simulink model "SM_FO_Simulink"  (R2025a)
settings: Solver=VariableStepAuto  StartTime=0.0  StopTime=10.0  RelTol=1e-3
settings Model: Creator=ryanjing  LastModifiedBy=ryanjing

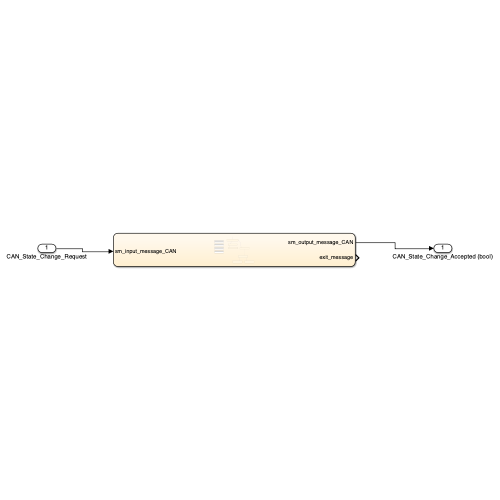
[thumbnail: Simulink's stored preview of the top-level diagram]
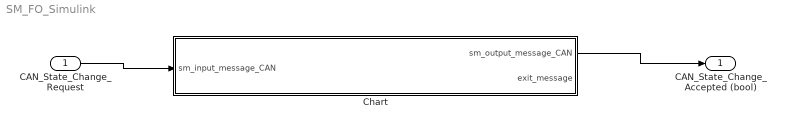
== system SM_FO_Simulink ==
  CAN_State_Change_Request : Inport
  Chart : Stateflow chart  TreatAsAtomicUnit=on
  CAN_State_Change_Accepted (bool) : Outport
  wires:
  CAN_State_Change_Request/1 -> Chart/1(sm_input_message_CAN)
  Chart/1(sm_output_message_CAN) -> CAN_State_Change_Accepted (bool)/1

== stateflow chart SM_FO_Simulink/Chart ==
  state Entry_State
    entry:
    parsed_message = parseCANMessage(sm_input_message_CAN);
  state Init_State
    entry:
    entry_status = SMFO_Init(sm_input_message_CAN);
  state Started_State
    entry:
    fprintf('Exit status: %f\n, vehicle started', entry_status)
    exit_message = entry_status;
  state Check_Message_State
    entry:
    state_request = GetCANMessage(parsed_message);
  state ACC_State
    entry:
    fprintf('ACC Requested')
    accAllowed = checkACCAllowed();
  state ACC_State1
    entry:
    fprintf('ACC Denied')
    sm_output_message_CAN = accAllowed;
  state ACC_State2
    entry:
    fprintf('ACC Accepted, sending ACC allow message');
    sm_output_message_CAN = accAllowed;
  (default) -> Entry_State
  Entry_State -> Check_Message_State [order 1] : [parsed_message > 0]
  Entry_State -> Init_State [order 2] : [parsed_message == 0]
  Init_State -> Started_State
  Check_Message_State -> ACC_State : [state_request == 2]
  ACC_State -> ACC_State1 [order 1] : [accAllowed == 0]
  ACC_State -> ACC_State2 [order 2] : [accAllowed == 1]
  data: input_CAN_data function_input; parsed_data function_output; input_CAN_data function_input; sm_status function_output; parsed_CAN_data function_input; message_request function_output; accAllowed function_output; sm_status local; sm_input_message_CAN input; entry_status local; accAllowed local; sm_output_message_CAN output; state_request local; parsed_message local; exit_message output
  function parsed_data = parseCANMessage(input_CAN_data):
    | function parsed_data = parseCANMessage(input_CAN_data)
    |     parsed_data = 1;
    | return
  function sm_status = SMFO_Init(input_CAN_data):
    | % enum off, standby, active, etc
    | function sm_status = SMFO_Init(input_CAN_data)
    |     InitializeStateMessages();
    |     sm_status_init = InitializeCarStructs(input_CAN_data);
    | 
    |     fprintf('State Machine status is: %f\n', sm_status_init);
    | 
    |     sm_status = sm_status_init;
    | 
    | end
    | 
    | function InitializeStateMessages()
    | 
    | end
    | 
    | function sm_status = InitializeCarStructs(input_CAN_data)
    |     carFeatureStatus = struct( ...
    |         'CACC', 0, ...
    |         'ACC', 0, ...
    |         'AIN', 0, ...
    |         'LCC', 0, ...
    |         'AP', 0 ...
    |     );
    | 
    |     carSwitches = struct(...
    |         'V2X', 0, ...
    |         'LongSwitch', 0, ...
    |         'LatSwitch', 0 ...  
    |     );
    | 
    |     carMainDriveInputs = struct(...
    |         'Speed', 0, ...
    |         'Brake_Pressed', 0 ...
    |     );
    | 
    |     carManualControlInputs = struct(...
    |         'Enable_ACC', 0, ...
    |         'Enable_AIN', 0, ...
    |         'Enable_CACC', 0, ...
    |         'Enable_LCC', 0, ...
    |         'Enable_AP', 0, ...
    |         'Cancel_Button', 0, ...
    |         'Set_Button', 0, ...
    |         'Finish_Button', 0 ...
    |     );
    | 
    |     carSensorInputs = struct(...
    |         'Lane_Detected', 0, ...
    |         'Parking_Space_Distance', 0, ...
    |         'Lane_Centered', 0 ...
    |     );
    | 
    |     overallCarStruct = struct( ...
    |         'FeatureStatus', carFeatureStatus, ...
    |         'Switches', carSwitches, ...
    |         'MainDriveInputs', carMainDriveInputs, ...
    |         'ManualControlInputs', carManualControlInputs, ...
    |         'SensorInputs', carSensorInputs ...
    |     );
    | 
    |     sm_status = 1;
    | 
    | end
  function message_request = GetCANMessage(parsed_CAN_data):
    | function message_request = GetCANMessage(parsed_CAN_data)
    |     if parsed_CAN_data > 0
    |         message_request = 2;
    |     else
    |         message_request = 0;
    |     end
    | end
  function accAllowed = checkACCAllowed:
    | function accAllowed = checkACCAllowed()
    |     % accAllowed = overallCarStruct.ManualControlInputs.EnableACC;
    |     accAllowed = 1;
    | end
